simulink model "gm_PN_generatorV2"  (R2020a)
settings: Solver=FixedStepDiscrete  StartTime=0.0  StopTime=20  RelTol=1e-3
undefined symbols (not defined in the file or in its folder): filt
libraries: commdigbbndpm3 x2, commfilt2 x2, commseqgen3 x2, dspmlti4 x2, commchan3 x1
settings Model: Creator=juanj  LastModifiedBy=juanj
settings OptimizationCC: BlockReduction=off  ConditionallyExecuteInputs=off  DefaultParameterBehavior=Inlined
settings DebuggingCC: AlgebraicLoopMsg=error  InheritedTsInSrcMsg=none  SingleTaskRateTransMsg=error
settings HardwareCC: ProdBitPerPointer=32  ProdBitPerSizeT=32  ProdBitPerPtrDiffT=32  ProdLargestAtomicFloat=None  ProdIntDivRoundTo=Undefined  ProdEndianess=Unspecified  ProdWordSize=32  ProdHWDeviceType=ASIC/FPGA->ASIC/FPGA  TargetBitPerPointer=64  TargetBitPerSizeT=64  TargetBitPerPtrDiffT=64  TargetLongLongMode=on  TargetIntDivRoundTo=Zero  TargetEndianess=LittleEndian  TargetWordSize=64  TargetHWDeviceType=Custom Processor->MATLAB Host Computer  ProdEqTarget=off

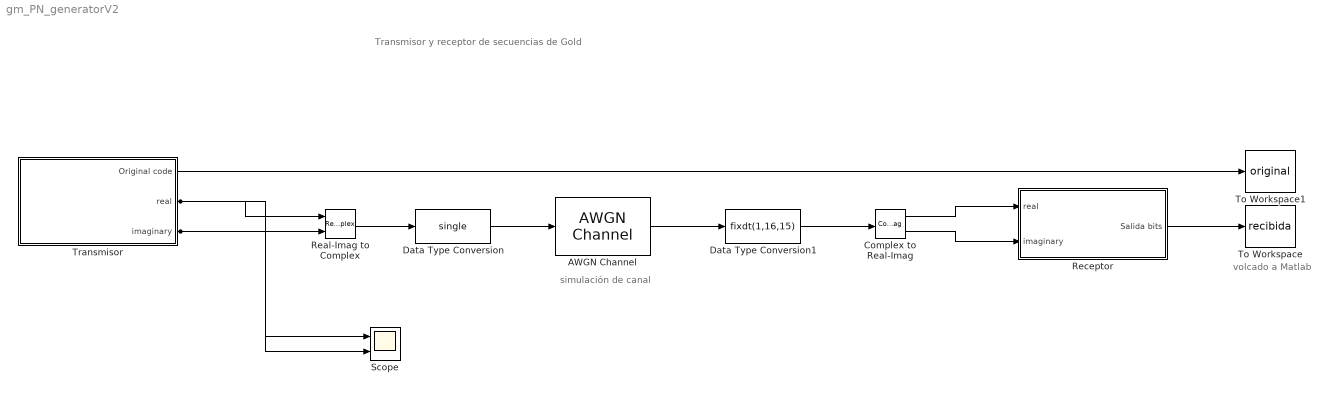
== system gm_PN_generatorV2 ==
  note: Transmisor y receptor de secuencias de Gold
  note: simulación de canal
  note: volcado a Matlab
  AWGN Channel : commchan3/AWGN Channel  InputProcessing=Columns as channels (frame based)  seed=67  noiseMode="Signal to noise ratio  (Es/No)"  EbNodB=10  EsNodB=10  SNRdB=10  bitsPerSym=1  Ps=1  Tsym=0.1  variance=1
  Complex to Real-Imag : ComplexToRealImag
  Data Type Conversion : DataTypeConversion  OutDataTypeStr=single
  Data Type Conversion1 : DataTypeConversion  OutDataTypeStr=fixdt(1,16,15)
  Real-Imag to Complex : RealImagToComplex
  Receptor : Subsystem  TreatAsAtomicUnit=on
  Scope : Scope  NumInputPorts=2
  To Workspace : ToWorkspace  VariableName=recibida  SampleTime=-1
      settings: Save2DSignal=2-D array (concatenate along first dimension)
  To Workspace1 : ToWorkspace  VariableName=original  SampleTime=-1
      settings: Save2DSignal=2-D array (concatenate along first dimension)
  Transmisor : Subsystem  TreatAsAtomicUnit=on
  wires:
  Transmisor/1(Original code) -> To Workspace1/1
  Data Type Conversion/1 -> AWGN Channel/1
  Data Type Conversion1/1 -> Complex to Real-Imag/1
  AWGN Channel/1 -> Data Type Conversion1/1
  Complex to Real-Imag/2 -> Receptor/2(imaginary)
  Complex to Real-Imag/1 -> Receptor/1(real)
  Transmisor/2(real) -> Real-Imag to Complex/1, Scope/1
  Transmisor/3(imaginary) -> Real-Imag to Complex/2, Scope/2
  Real-Imag to Complex/1 -> Data Type Conversion/1
  Receptor/1(Salida bits) -> To Workspace/1

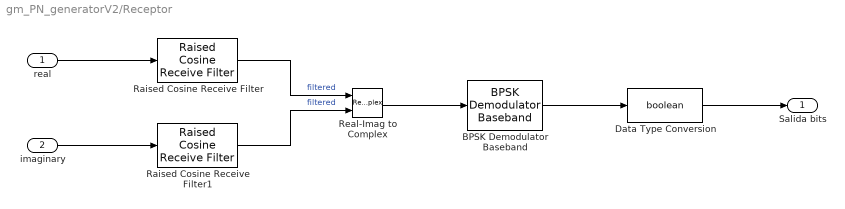
== system gm_PN_generatorV2/Receptor ==
  real : Inport
  imaginary : Inport  Port=2
  BPSK Demodulator Baseband : commdigbbndpm3/BPSK Demodulator Baseband  DecType=Hard decision  VarSource=Dialog  Variance=1  Ph=0  outDtype=Inherit via internal rule  derotateFactorWordLen=16  derotateFactorDataTypeStr=Inherit: Same word length as input  derotateFactorLastDataTypeStr=Inherit: Same word length as input
  Data Type Conversion : DataTypeConversion  OutDataTypeStr=boolean
  Raised Cosine Receive Filter : commfilt2/Raised Cosine Receive Filter  filtType=Square root  R=0.5  filtSpan=16  N=16  downFactor=16  downOffset=0  filterGain=2  RateOptions=Allow multirate processing  framing=Mute  checkCoeff=off  variableName=rcRxFilt  currentFiltSpan=16  D=(16)/2  inputOffset=0  sampMode=Mute  saveAsFlag=0  rateMode=Downsampling  checkGain=Normalized  launchFVT=on  roundingMode=Floor  overflowMode=off  coeffDataTypeStr=Inherit: Same word length as input  coeffMin=[]  coeffMax=[]  coeffLastDataTypeStr=Inherit: Same word length as input  accumDataTypeStr=Inherit: Same as product output  accumLastDataTypeStr=Inherit: Same as product output  outputDataTypeStr=Inherit: Same as accumulator  outputMin=[]  outputMax=[]  outputLastDataTypeStr=Inherit: Same as accumulator
  Raised Cosine Receive Filter1 : commfilt2/Raised Cosine Receive Filter  filtType=Square root  R=0.5  filtSpan=16  N=16  downFactor=16  downOffset=0  filterGain=2  RateOptions=Allow multirate processing  framing=Mute  checkCoeff=off  variableName=rcRxFilt1  currentFiltSpan=16  D=(16)/2  inputOffset=0  sampMode=Mute  saveAsFlag=0  rateMode=Downsampling  checkGain=Normalized  launchFVT=on  roundingMode=Floor  overflowMode=off  coeffDataTypeStr=Inherit: Same word length as input  coeffMin=[]  coeffMax=[]  coeffLastDataTypeStr=Inherit: Same word length as input  accumDataTypeStr=Inherit: Same as product output  accumLastDataTypeStr=Inherit: Same as product output  outputDataTypeStr=Inherit: Same as accumulator  outputMin=[]  outputMax=[]  outputLastDataTypeStr=Inherit: Same as accumulator
  Real-Imag to Complex : RealImagToComplex
  Salida bits : Outport
  wires:
  Data Type Conversion/1 -> Salida bits/1
  real/1 -> Raised Cosine Receive Filter/1
  Real-Imag to Complex/1 -> BPSK Demodulator Baseband/1
  Raised Cosine Receive Filter1/1 -> Real-Imag to Complex/2  "filtered"
  imaginary/1 -> Raised Cosine Receive Filter1/1
  BPSK Demodulator Baseband/1 -> Data Type Conversion/1
  Raised Cosine Receive Filter/1 -> Real-Imag to Complex/1  "filtered"

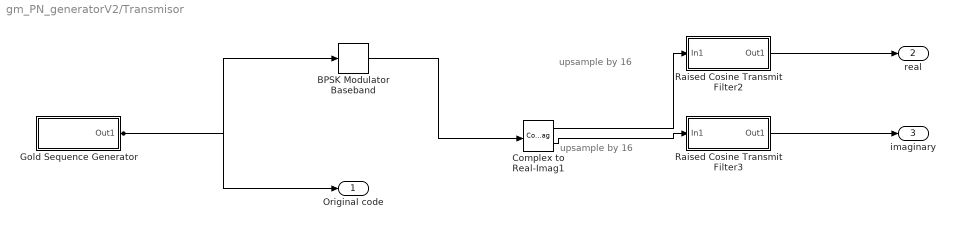
== system gm_PN_generatorV2/Transmisor ==
  note: upsample by 16
  note: upsample by 16
  BPSK Modulator Baseband : commdigbbndpm3/BPSK Modulator Baseband  Ph=0  outDtype=Fixed-point  outWordLen=16  outUDDataType=sfix(16)  outFracLenMode=Best precision  outFracLen=15  outDataTypeStr=fixdt(1,16)  outLastDataTypeStr=fixdt(1,16)
  Complex to Real-Imag1 : ComplexToRealImag  SampleTime=0.01
  Gold Sequence Generator : Subsystem  mask(Gold Sequence Generator){genPoly1='z^6 + z + 1', iniState1=[0 1 0 1 0 1], genPoly2='z^6 + z^5 + z^2 + z + 1', iniState2=[0 0 0 0 0 1], index=double(0), shift=double(0), outVarSiz=off, maxOutSizeMode=Dialog parameter, maxOutSize=[10 1], Ts=1/100, sampPerFrame=1, reset=off, outDataType=boolean}
      mask prompts: genPoly1 "Preferred polynomial (1):"; iniState1 "Initial states (1):"; genPoly2 "Preferred polynomial (2):"; iniState2 "Initial states (2):"; index "Sequence index:"; outVarSiz "Output variable-size signals"; maxOutSizeMode "Maximum output size source:"; maxOutSize "Maximum output size:"; Ts "Sample time:"; sampPerFrame "Samples per frame:"; reset "Reset on nonzero input"; outDataType "Output data type:"
      mask help:
      | Generate a Gold sequence from a set of sequences by specifying a preferred pair of polynomials.
      |
      | The polynomial parameter values represent the shift register connections. Enter these values as either a polynomial string, a binary vector or a descending ordered polynomial to indicate the connection points.
      |
      | The sequence index parameter denotes the single sequence outputted from the set of Gold sequences. Specify it as a scalar integer in the range [-2, 2^n-2] where n is the degree of the generator polynomial. The index values -2 and -1 correspond to the first and second PN sequences as generated by the preferred polynomials (1) and (2), respectively.
      |
      | For variable-size output signals, the current output size is either specified from the 'oSiz' input or inherited from the 'Ref' input.
      mask init:
      | [eStr, genPoly1, iniState1, genPoly2, iniState2, index, shift] = commblkgcgen3(gcb, 'init', genPoly1, iniState1, genPoly2, iniState2, shift, index, sampPerFrame);
      | if (eStr.ecode == 1)
      | 	error(eStr.eID, eStr.emsg);
      | end
      | % Initial states are from the dialog always
      | iniStaSource = 1;
      mask Help: eval('blocksethelp');
      mask Callback outVarSiz: commblkgcgen3(gcb, 'cbvarsize');
      mask TypeOptions maxOutSizeMode: Dialog parameter | Inherit from reference input
      mask Callback maxOutSizeMode: commblkgcgen3(gcb,'cbmaxoutsrc');
      mask TypeOptions outDataType: double | boolean | Smallest unsigned integer
      mask Callback outDataType: commblkgcgen3(gcb,'cbOutDType');
      mask Display:
      | disp('Gold Sequence\nGenerator');
      | 
      | % Port Labels (alongwith location in normalized units)
      | vSizPortLbl.str = ''; vSizPortLbl.x = 0.0; vSizPortLbl.y = 0.0;
      | rstPortLbl.str = ''; rstPortLbl.x = 0.0; rstPortLbl.y = 0.0;
      | 
      | % Oriented positions (in normalized units) for ONLY ONE INPUT PORT
      | xRightOneInport = 0.03; yRightOneInport = 0.5;
      | xLeft_OneInport = 0.82; yLeft_OneInport = 0.5;
      | xUp___OneInport = 0.5; yUp___OneInport = 0.05;
      | xDown_OneInport = 0.5; yDown_OneInport = 0.93;
      | 
      | % Oriented positions (in normalized units) for TWO INPUT PORTS
      | xRightInport1 = 0.03; yRightInport1 = 0.75;
      | xRightInport2 = 0.03; yRightInport2 = 0.25;
      | xLeft_Inport1 = 0.82; yLeft_Inport1 = 0.75;
      | xLeft_Inport2 = 0.82; yLeft_Inport2 = 0.25;
      | xUp___Inport1 = 0.25; yUp___Inport1 = 0.05;
      | xUp___Inport2 = 0.75; yUp___Inport2 = 0.05;
      | xDown_Inport1 = 0.25; yDown_Inport1 = 0.93;
      | xDown_Inport2 = 0.75; yDown_Inport2 = 0.93;
      | 
      | blkOrientationStr = lower(get_param(gcbh, 'orientation'));
      | 
      | if (outVarSiz==0)
      |     if (reset==1) % only reset
      |         rstPortLbl.str = 'Rst';
      |         switch blkOrientationStr
      |             case 'right'
      |                 rstPortLbl.x = xRightOneInport;
      |                 rstPortLbl.y = yRightOneInport;
      |             case 'left'
      |                 rstPortLbl.x = xLeft_OneInport;
      |                 rstPortLbl.y = yLeft_OneInport;
      |             case 'up'
      |                 rstPortLbl.x = xUp___OneInport;
      |                 rstPortLbl.y = yUp___OneInport;
      |             otherwise % down
      |                 rstPortLbl.x = xDown_OneInport;
      |                 rstPortLbl.y = yDown_OneInport;
      |         end
      |     end
      | else % vSiz port on
      |     if (maxOutSizeMode==1)
      |        vSizPortLbl.str = 'oSiz';
      |     else
      |         vSizPortLbl.str = 'Ref';
      |     end
      |     if (reset==1) % both
      |         rstPortLbl.str = 'Rst';
      |         switch blkOrientationStr
      |             case 'right'
      |                 vSizPortLbl.x = xRightInport1;
      |                 vSizPortLbl.y = yRightInport1;
      |                 rstPortLbl.x = xRightInport2;
      |                 rstPortLbl.y = yRightInport2;
      |             case 'left'
      |                 vSizPortLbl.x = xLeft_Inport1;
      |                 vSizPortLbl.y = yLeft_Inport1;
      |                 rstPortLbl.x = xLeft_Inport2;
      |                 rstPortLbl.y = yLeft_Inport2;
      |             case 'up'
      |                 vSizPortLbl.x = xUp___Inport1;
      |                 vSizPortLbl.y = yUp___Inport1;
      |                 rstPortLbl.x = xUp___Inport2;
      |                 rstPortLbl.y = yUp___Inport2;
      |             otherwise % down
      |                 vSizPortLbl.x = xDown_Inport1;
      |                 vSizPortLbl.y = yDown_Inport1;
      |                 rstPortLbl.x = xDown_Inport2;
      |                 rstPortLbl.y = yDown_Inport2;
      |         end
      |     else % no reset, vSiz only
      |         switch blkOrientationStr
      |             case 'right'
      |                 vSizPortLbl.x = xRightOneInport;
      |                 vSizPortLbl.y = yRightOneInport;
      |             case 'left'
      |                 vSizPortLbl.x = xLeft_OneInport;
      |                 vSizPortLbl.y = yLeft_OneInport;
      |             case 'up'
      |                 vSizPortLbl.x = xUp___OneInport;
      |                 vSizPortLbl.y = yUp___OneInport;
      |             otherwise
      |                 vSizPortLbl.x = xDown_OneInport;
      |                 vSizPortLbl.y = yDown_OneInport;
      |         end
      |     end
      | end
      | 
      | text(vSizPortLbl.x, vSizPortLbl.y, vSizPortLbl.str);
      | text(rstPortLbl.x, rstPortLbl.y, rstPortLbl.str);
  Raised Cosine Transmit Filter2 : Subsystem  mask(Raised Cosine Transmit Filter){filtType=Square root, R=double(0.5), filtSpan=double(16), N=double(16), filterGain=double(2), InputProcessing=Elements as channels (sample based), RateOptions=Allow multirate processing, framing=Mute, checkCoeff=off, variableName=rcTxFilt2, checkGain=Normalized, sampMode=Mute, saveAsFlag=double(0), currentFiltSpan=double(16), D=double(8), launchFVT=on, roundingMode=Floor, overflowMode=off, coeffMode=Same word length as input, coeffWordLength=double(16), coeffFracLength=double(15), coeffDataTypeStr=Inherit: Same word length as input, coeffMin=[], coeffMax=[], coeffLastDataTypeStr=Inherit: Same word length as input, prodOutputMode=Inherit via internal rule, prodOutputWordLength=double(32), prodOutputFracLength=double(30), prodOutputDataTypeStr=Inherit: Inherit via internal rule, prodOutputLastDataTypeStr=Inherit: Inherit via internal rule, accumMode=Inherit via internal rule, accumWordLength=double(32), accumFracLength=double(30), accumDataTypeStr=Inherit: Inherit via internal rule, accumLastDataTypeStr=Inherit: Inherit via internal rule, outputMode=Same as input, outputWordLength=double(16), outputFracLength=double(15), outputDataTypeStr=Inherit: Same as input, outputMin=[], outputMax=[], outputLastDataTypeStr=Inherit: Same as input, LockScale=off}
      mask prompts: filtType "Filter shape:"; R "Rolloff factor:"; filtSpan "Filter span in symbols:"; N "Output samples per symbol:"; filterGain "Linear amplitude filter gain:"; InputProcessing "dsp:FIRMultirateBlockDialog:InputProc_MP"; RateOptions "dsp:FIRMultirateBlockDialog:RateOptions_MP"; checkCoeff "Export filter coefficients to workspace"; variableName "Coefficient variable name:"; checkGain "Filter gain:"; sampMode "Input sampling mode:"; saveAsFlag "Save_as flag:"; currentFiltSpan "Current filter span in symbols:"; D "Group delay (number of symbols):"; launchFVT "Visualize filter with FVTool"; roundingMode "dspshared:FixptDialog:roundingMode"; overflowMode "Simulink:masks:SaturateOnIntegerOverflow_MP"; LockScale "dspshared:FixptDialog:lockAgnstChanges"
      mask help: Upsample and filter the input signal using a normal or square root raised cosine FIR filter.
      mask init:
      | commblkrcfilttx(gcbh,'frameupgrademultirate');
      | 
      | [filt, icon, err] = commblkrcfilttx(gcbh,'init',...
      |     filtType, R, filtSpan, currentFiltSpan, D, N, filterGain, ...
      |     checkCoeff, variableName);
      | 
      | % Set sample modes of underlying blocks
      | commblkrcfilttx(gcb,'setFIRInterp', InputProcessing, RateOptions, ...
      |     roundingMode, overflowMode, LockScale);
      | 
      | if(~isempty(err.msg))
      | 	error(err.eID,err.msg);
      | end
      mask Help: eval('blocksethelp');
      mask TypeOptions filtType: Normal | Square root
      mask TypeOptions InputProcessing: Columns as channels (frame based) | Elements as channels (sample based)
      mask Callback InputProcessing: commblkrcfilttx(gcbh,'cbInputProcessing');
      mask TypeOptions RateOptions: Enforce single-rate processing | Allow multirate processing
      mask TypeOptions framing: Enforce single-rate processing | Allow multirate processing | Maintain input frame rate | Maintain input frame size | Mute
      mask Callback checkCoeff: commblkrcfilttx(gcbh,'cbCheckCoeff');
      mask Callback variableName: commblkrcfilttx(gcbh,'dialogdynamic');
      mask TypeOptions checkGain: Normalized | User-specified
      mask TypeOptions sampMode: Frame-based | Sample-based | Mute
      mask TypeOptions roundingMode: Ceiling | Convergent | Floor | Nearest | Round | Simplest | Zero
      mask TypeOptions coeffMode: Same word length as input | Specify word length | Binary point scaling | Slope and bias scaling
      mask TypeOptions prodOutputMode: Inherit via internal rule | Same as input | Binary point scaling | Slope and bias scaling
      mask TypeOptions accumMode: Inherit via internal rule | Same as product output | Same as input | Binary point scaling | Slope and bias scaling
      mask TypeOptions outputMode: Same as accumulator | Same as product output | Same as input | Binary point scaling | Slope and bias scaling
      mask Display:
      | plot(0,0,1,1,icon.xx,icon.plot);
      | text(icon.x,icon.y,icon.str,'horiz','center');
  Raised Cosine Transmit Filter3 : Subsystem  mask(Raised Cosine Transmit Filter){filtType=Square root, R=double(0.5), filtSpan=double(16), N=double(16), filterGain=double(2), InputProcessing=Elements as channels (sample based), RateOptions=Allow multirate processing, framing=Mute, checkCoeff=off, variableName=rcTxFilt3, checkGain=Normalized, sampMode=Mute, saveAsFlag=double(0), currentFiltSpan=double(16), D=double(8), launchFVT=on, roundingMode=Floor, overflowMode=off, coeffMode=Same word length as input, coeffWordLength=double(16), coeffFracLength=double(15), coeffDataTypeStr=Inherit: Same word length as input, coeffMin=[], coeffMax=[], coeffLastDataTypeStr=Inherit: Same word length as input, prodOutputMode=Inherit via internal rule, prodOutputWordLength=double(32), prodOutputFracLength=double(30), prodOutputDataTypeStr=Inherit: Inherit via internal rule, prodOutputLastDataTypeStr=Inherit: Inherit via internal rule, accumMode=Inherit via internal rule, accumWordLength=double(32), accumFracLength=double(30), accumDataTypeStr=Inherit: Inherit via internal rule, accumLastDataTypeStr=Inherit: Inherit via internal rule, outputMode=Same as input, outputWordLength=double(16), outputFracLength=double(15), outputDataTypeStr=Inherit: Same as input, outputMin=[], outputMax=[], outputLastDataTypeStr=Inherit: Same as input, LockScale=off}
      mask prompts: filtType "Filter shape:"; R "Rolloff factor:"; filtSpan "Filter span in symbols:"; N "Output samples per symbol:"; filterGain "Linear amplitude filter gain:"; InputProcessing "dsp:FIRMultirateBlockDialog:InputProc_MP"; RateOptions "dsp:FIRMultirateBlockDialog:RateOptions_MP"; checkCoeff "Export filter coefficients to workspace"; variableName "Coefficient variable name:"; checkGain "Filter gain:"; sampMode "Input sampling mode:"; saveAsFlag "Save_as flag:"; currentFiltSpan "Current filter span in symbols:"; D "Group delay (number of symbols):"; launchFVT "Visualize filter with FVTool"; roundingMode "dspshared:FixptDialog:roundingMode"; overflowMode "Simulink:masks:SaturateOnIntegerOverflow_MP"; LockScale "dspshared:FixptDialog:lockAgnstChanges"
      mask help: Upsample and filter the input signal using a normal or square root raised cosine FIR filter.
      mask init: same as gm_PN_generatorV2/Transmisor/Raised Cosine Transmit Filter2
      mask Help: eval('blocksethelp');
      mask TypeOptions filtType: Normal | Square root
      mask TypeOptions InputProcessing: Columns as channels (frame based) | Elements as channels (sample based)
      mask Callback InputProcessing: commblkrcfilttx(gcbh,'cbInputProcessing');
      mask TypeOptions RateOptions: Enforce single-rate processing | Allow multirate processing
      mask TypeOptions framing: Enforce single-rate processing | Allow multirate processing | Maintain input frame rate | Maintain input frame size | Mute
      mask Callback checkCoeff: commblkrcfilttx(gcbh,'cbCheckCoeff');
      mask Callback variableName: commblkrcfilttx(gcbh,'dialogdynamic');
      mask TypeOptions checkGain: Normalized | User-specified
      mask TypeOptions sampMode: Frame-based | Sample-based | Mute
      mask TypeOptions roundingMode: Ceiling | Convergent | Floor | Nearest | Round | Simplest | Zero
      mask TypeOptions coeffMode: Same word length as input | Specify word length | Binary point scaling | Slope and bias scaling
      mask TypeOptions prodOutputMode: Inherit via internal rule | Same as input | Binary point scaling | Slope and bias scaling
      mask TypeOptions accumMode: Inherit via internal rule | Same as product output | Same as input | Binary point scaling | Slope and bias scaling
      mask TypeOptions outputMode: Same as accumulator | Same as product output | Same as input | Binary point scaling | Slope and bias scaling
      mask Display:
      | plot(0,0,1,1,icon.xx,icon.plot);
      | text(icon.x,icon.y,icon.str,'horiz','center');
  Original code : Outport
  real : Outport  Port=2
  imaginary : Outport  Port=3
  wires:
  BPSK Modulator Baseband/1 -> Complex to Real-Imag1/1
  Complex to Real-Imag1/1 -> Raised Cosine Transmit Filter2/1(In1)
  Complex to Real-Imag1/2 -> Raised Cosine Transmit Filter3/1(In1)
  Gold Sequence Generator/1(Out1) -> Original code/1, BPSK Modulator Baseband/1
  Raised Cosine Transmit Filter2/1(Out1) -> real/1
  Raised Cosine Transmit Filter3/1(Out1) -> imaginary/1

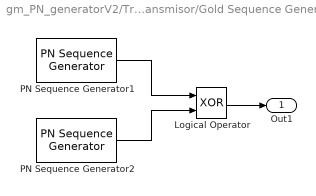
== system gm_PN_generatorV2/Transmisor/Gold Sequence Generator ==
  Logical Operator : Logic  Operator=XOR  AllPortsSameDT=off  OutDataTypeStr=boolean
  PN Sequence Generator1 : commseqgen3/PN Sequence Generator  poly=genPoly1  ini_sta=iniState1  outBitMaskSource=Dialog parameter  shift=shift  outVarSiz=off  maxOutSizeMode=Dialog parameter  maxOutSize=maxOutSize  Ts=Ts  sampPerFrame=sampPerFrame  reset=off  bitPackedOutputs=off  outDataType=boolean  numPackedBits=8  bitPackDataSigned=off  bitPackedOutDType=double
  PN Sequence Generator2 : commseqgen3/PN Sequence Generator  poly=genPoly2  ini_sta=iniState2  outBitMaskSource=Dialog parameter  shift=shift + index  outVarSiz=off  maxOutSizeMode=Dialog parameter  maxOutSize=maxOutSize  Ts=Ts  sampPerFrame=sampPerFrame  reset=off  bitPackedOutputs=off  outDataType=boolean  numPackedBits=8  bitPackDataSigned=off  bitPackedOutDType=double
  Out1 : Outport
  wires:
  Logical Operator/1 -> Out1/1
  PN Sequence Generator1/1 -> Logical Operator/1
  PN Sequence Generator2/1 -> Logical Operator/2

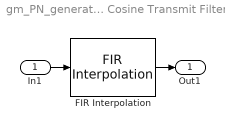
== system gm_PN_generatorV2/Transmisor/Raised Cosine Transmit Filter2 ==
  In1 : Inport  OutDataTypeStr=fixdt(1, 16, 15)  SampleTime=0.01
  FIR Interpolation : dspmlti4/FIR Interpolation  FilterSource=Dialog parameters  PrivateCoeffs=0  h=filt.coeff  L=filt.rateFactor  FilterObject=Hm_firinterp  framing=Allow multirate processing  outputBufInitCond=0  roundingMode=Floor  overflowMode=off  firstCoeffDataTypeStr=Inherit: Same word length as input  firstCoeffMin=[]  firstCoeffMax=[]  firstCoeffLastDataTypeStr=Inherit: Same word length as input  outputMin=[]  outputMax=[]
  Out1 : Outport
  wires:
  In1/1 -> FIR Interpolation/1
  FIR Interpolation/1 -> Out1/1

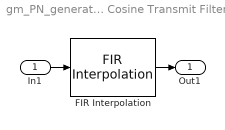
== system gm_PN_generatorV2/Transmisor/Raised Cosine Transmit Filter3 ==
  In1 : Inport  OutDataTypeStr=fixdt(1, 16, 15)  SampleTime=0.01
  FIR Interpolation : dspmlti4/FIR Interpolation  FilterSource=Dialog parameters  PrivateCoeffs=0  h=filt.coeff  L=filt.rateFactor  FilterObject=Hm_firinterp  framing=Allow multirate processing  outputBufInitCond=0  roundingMode=Floor  overflowMode=off  firstCoeffDataTypeStr=Inherit: Same word length as input  firstCoeffMin=[]  firstCoeffMax=[]  firstCoeffLastDataTypeStr=Inherit: Same word length as input  outputMin=[]  outputMax=[]
  Out1 : Outport
  wires:
  In1/1 -> FIR Interpolation/1
  FIR Interpolation/1 -> Out1/1
